simulink model "cessna172_model"  (R2024a)
settings: Solver=VariableStepAuto  StartTime=0.0  StopTime=60  RelTol=1e-9
settings Model: Creator=sundharvs  LastModifiedBy=sundhar
settings DataIOCC: SaveState=on  SignalLogging=off  DSMLogging=off  ReturnWorkspaceOutputs=off
settings RTWCC: GPUComputeCapability=3.5

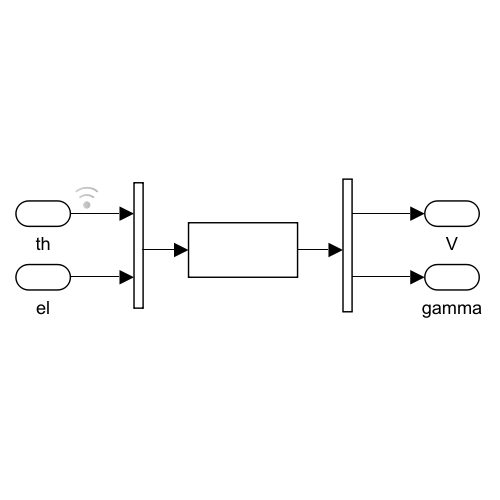
[thumbnail: Simulink's stored preview of the top-level diagram]
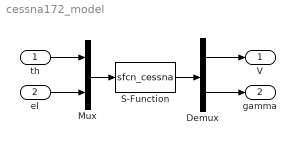
== system cessna172_model ==
  th : Inport
  el : Inport  Port=2
  Demux : Demux  Outputs=2
  Mux : Mux  Inputs=2
  S-Function : S-Function  FunctionName=sfcn_cessna  SFunctionDeploymentMode=off  EnableBusSupport=off
  V : Outport
  gamma : Outport  Port=2
  wires:
  Mux/1 -> S-Function/1
  th/1 -> Mux/1
  el/1 -> Mux/2
  S-Function/1 -> Demux/1
  Demux/1 -> V/1
  Demux/2 -> gamma/1
